simulink model "test6_namechange_diff"  (R2018a)
settings: Solver=VariableStepAuto  StartTime=0.0  StopTime=10.0  RelTol=1e-3
settings Model: Creator=monika  LastModifiedBy=monika

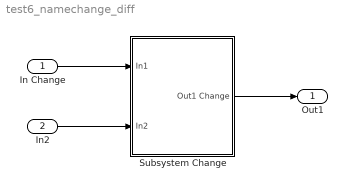
== system test6_namechange_diff ==
  In Change : Inport
  In2 : Inport  Port=2
  Subsystem Change : Subsystem
  Out1 : Outport
  wires:
  In2/1 -> Subsystem Change/2(In2)
  In Change/1 -> Subsystem Change/1(In1)
  Subsystem Change/1(Out1 Change) -> Out1/1

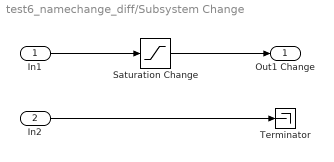
== system test6_namechange_diff/Subsystem Change ==
  In1 : Inport
  In2 : Inport  Port=2
  Saturation Change : Saturate
  Terminator : Terminator
  Out1 Change : Outport
  wires:
  In2/1 -> Terminator/1
  In1/1 -> Saturation Change/1
  Saturation Change/1 -> Out1 Change/1
